simulink model "testYarpSendBML_stateflow"  (R2014a)
settings: Solver=FixedStepDiscrete  StartTime=0.0  StopTime=20  FixedStep=0.0002  RelTol=1e-3
model workspace (MAT data in the model file):
  gtest = 0
settings Model: Creator=Ulysses  LastModifiedBy=Ulysses

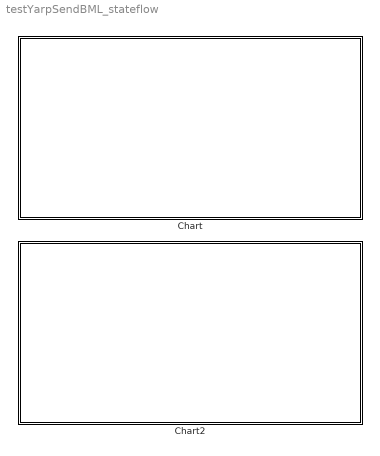
== system testYarpSendBML_stateflow ==
  Chart : Stateflow chart  TreatAsAtomicUnit=on
  Chart2 : Stateflow chart  TreatAsAtomicUnit=on

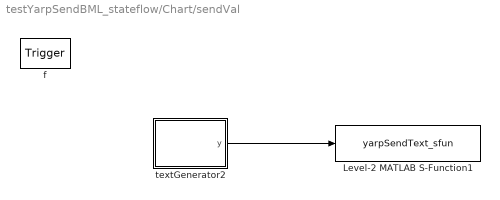
== system testYarpSendBML_stateflow/Chart/sendVal ==
  f : TriggerPort  TriggerType=function-call
      settings: CopyFcn=Stateflow.SLINSF.SimulinkMan.removeBlockPreDeleteFcn  PreDeleteFcn=Stateflow.SLINSF.SimulinkMan.unsafePredeleteFcn
  Level-2 MATLAB S-Function1 : M-S-Function  FunctionName=yarpSendText_sfun  Parameters='/sim/out/smb', '/rs'
  textGenerator2 : MATLAB Function  TreatAsAtomicUnit=on
  wires:
  textGenerator2/1(y) -> Level-2 MATLAB S-Function1/1

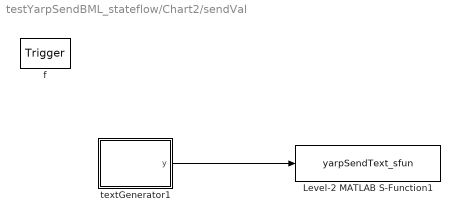
== system testYarpSendBML_stateflow/Chart2/sendVal ==
  f : TriggerPort  TriggerType=function-call
      settings: CopyFcn=Stateflow.SLINSF.SimulinkMan.removeBlockPreDeleteFcn  PreDeleteFcn=Stateflow.SLINSF.SimulinkMan.unsafePredeleteFcn
  Level-2 MATLAB S-Function1 : M-S-Function  FunctionName=yarpSendText_sfun  Parameters='/sim/out/bml', '/rr'
  textGenerator1 : MATLAB Function  TreatAsAtomicUnit=on
  wires:
  textGenerator1/1(y) -> Level-2 MATLAB S-Function1/1

== stateflow chart testYarpSendBML_stateflow/Chart2 ==
  state state02
    entry: sendVal()
  state state01
    entry: sendVal()
  state sendVal [function]
  (default) -> state01
  state01 -> state02 : after(2,sec)
  state02 -> state01 : after(2,sec)

== matlab function testYarpSendBML_stateflow/Chart2/sendVal/textGenerator1 ==
  data: y output
function y = fcn()
y = encStr2Arr('test string 2');

== stateflow chart testYarpSendBML_stateflow/Chart ==
  state state02
    entry: sendVal()
  state state01
    entry: sendVal()
  state sendVal [function]
  (default) -> state01
  state01 -> state02 : after(2,sec)
  state02 -> state01 : after(2,sec)

== matlab function testYarpSendBML_stateflow/Chart/sendVal/textGenerator2 ==
  data: y output
function y = fcn()
y = encStr2Arr('test string');
